simulink model "power"  (R2021a)
settings: Solver=VariableStepAuto  StartTime=0.0  StopTime=Torb  RelTol=1e-3
values from neighbouring files (symbols this model uses):
  inc = 97.5*pi/180    (= 1.70169602069)    [params_power.m]
libraries: sharedtransform x12, aerolibutil x4
settings Model: Creator=Laura  LastModifiedBy=Laura

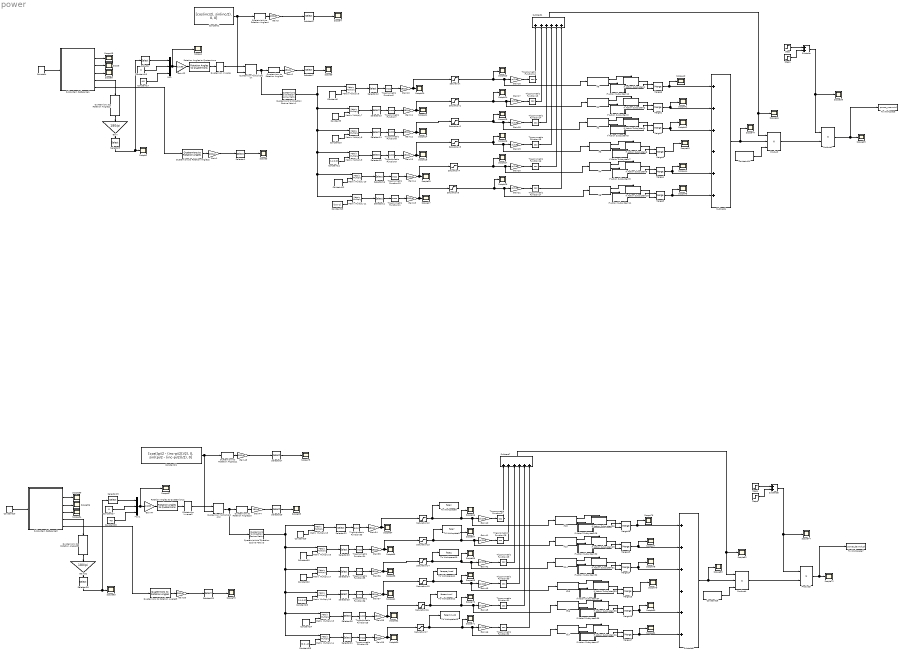
== system power ==
  Constant : Constant  Value=[0,0,0]
  Constant1 : Constant  Value=[cos(inc/2), sin(inc/2), 0, 0]
  Constant10 : Constant  Value=[0,0,1]
  Constant11 : Constant  Value=[-1,0,0]
  Constant12 : Constant  Value=[0,-1,0]
  Constant13 : Constant  Value=[0,0,-1]
  Constant14 : Constant  Value=1367*0.9*0.32*0.77
  Constant15 : Constant  Value=0
  Constant17 : Constant  Value=-45
  Constant20 : Constant  Value=[0,0,0]
  Constant21 : Constant  Value=[cos((pi/2 - (inc-pi/2))/2), 0, sin((pi/2 - (inc-pi/2))/2), 0]
  Constant22 : Constant  Value=[0,0,1]
  Constant23 : Constant  Value=[-1,0,0]
  Constant24 : Constant  Value=[0,-1,0]
  Constant25 : Constant  Value=[0,0,-1]
  Constant26 : Constant  Value=1367*0.9*0.32*0.77
  Constant27 : Constant  Value=0
  Constant28 : Constant  Value=-45
  Constant29 : Constant  Value=[1,0,0]
  Constant30 : Constant  Value=[0,1,0]
  Constant8 : Constant  Value=[1,0,0]
  Constant9 : Constant  Value=[0,1,0]
  Gain{,1..3,10..15,32..39,44,48} (20 alike) : Gain  Gain=180/pi
  Gain{16..22,40..43,45..47} (14 alike) : Gain  Gain=pi/180
  If Action Subsystem1 : Subsystem  TreatAsAtomicUnit=on
  If Action Subsystem10 : Subsystem  TreatAsAtomicUnit=on
  If Action Subsystem11 : Subsystem  TreatAsAtomicUnit=on
  If Action Subsystem12 : Subsystem  TreatAsAtomicUnit=on
  If Action Subsystem2 : Subsystem  TreatAsAtomicUnit=on
  If Action Subsystem25 : Subsystem  TreatAsAtomicUnit=on
  If Action Subsystem26 : Subsystem  TreatAsAtomicUnit=on
  If Action Subsystem27 : Subsystem  TreatAsAtomicUnit=on
  If Action Subsystem28 : Subsystem  TreatAsAtomicUnit=on
  If Action Subsystem29 : Subsystem  TreatAsAtomicUnit=on
  If Action Subsystem3 : Subsystem  TreatAsAtomicUnit=on
  If Action Subsystem30 : Subsystem  TreatAsAtomicUnit=on
  If Action Subsystem31 : Subsystem  TreatAsAtomicUnit=on
  If Action Subsystem32 : Subsystem  TreatAsAtomicUnit=on
  If Action Subsystem33 : Subsystem  TreatAsAtomicUnit=on
  If Action Subsystem34 : Subsystem  TreatAsAtomicUnit=on
  If Action Subsystem35 : Subsystem  TreatAsAtomicUnit=on
  If Action Subsystem36 : Subsystem  TreatAsAtomicUnit=on
  If Action Subsystem4 : Subsystem  TreatAsAtomicUnit=on
  If Action Subsystem5 : Subsystem  TreatAsAtomicUnit=on
  If Action Subsystem6 : Subsystem  TreatAsAtomicUnit=on
  If Action Subsystem7 : Subsystem  TreatAsAtomicUnit=on
  If Action Subsystem8 : Subsystem  TreatAsAtomicUnit=on
  If Action Subsystem9 : Subsystem  TreatAsAtomicUnit=on
  If{1..6,13..18} (12 alike) : If  IfExpression=u1 < 89.995
  Matrix Multiply{6..11,13..18} (12 alike) : Product  Multiplication=Matrix(*)
  Merge{1..6,13..18} (12 alike) : Merge
  Mux : Mux  Inputs=3
  Mux1 : Mux  Inputs=3
  Product : Product  Inputs=3
  Product1 : Product
  Product4 : Product  Inputs=3
  Product5 : Product
  Quaternion Inverse : aerolibutil/Quaternion Inverse
  Quaternion Inverse2 : aerolibutil/Quaternion Inverse
  Quaternion Multiplication : aerolibutil/Quaternion Multiplication
  Quaternion Multiplication2 : aerolibutil/Quaternion Multiplication
  Quaternions to Direction Cosine Matrix1 : sharedtransform/Quaternions to  Direction Cosine Matrix  aMode=aMode
      settings: SourceProductBaseCode=AE,PW,DR,MT,UV,VE
  Quaternions to Direction Cosine Matrix3 : sharedtransform/Quaternions to  Direction Cosine Matrix  aMode=aMode
      settings: SourceProductBaseCode=AE,PW,DR,MT,UV,VE
  Quaternions to Rotation Angles{1..5,9..11} (8 alike) : sharedtransform/Quaternions to Rotation Angles  rotationOrder=ZYX  aMode=aMode
      settings: SourceProductBaseCode=AE,PW,DR,MT,UV,VE
  Rotation Angles to Quaternions : sharedtransform/Rotation Angles to Quaternions  rotationOrder=ZYX  aMode=aMode
      settings: SourceProductBaseCode=AE,PW,DR,MT,UV,VE
  Rotation Angles to Quaternions1 : sharedtransform/Rotation Angles to Quaternions  rotationOrder=ZYX  aMode=aMode
      settings: SourceProductBaseCode=AE,PW,DR,MT,UV,VE
  Saturation{,1..5,12..17} (12 alike) : Saturate  UpperLimit=90.00005  LowerLimit=-90.00005
  Scope{,1..4,8..9,14..15,17..21,23..29,39..47,56..85} (60 alike) : Scope
  Selector : Selector  InputPortWidth=3  IndexOptions=Index vector (dialog)  Indices=[3]  OutputSizes=1
  Selector{1..3,7,20,27..29} (8 alike) : Selector  InputPortWidth=3  IndexOptions=Index vector (dialog)  Indices=[3 2 1]  OutputSizes=1
  Selector{11..16,21..26} (12 alike) : Selector  InputPortWidth=3  IndexOptions=Index vector (dialog)  Indices=[1]  OutputSizes=1
  Selector19 : Selector  InputPortWidth=3  IndexOptions=Index vector (dialog)  Indices=[3]  OutputSizes=1
  Step : Step  Time=30.76*60  Before=1  After=0  SampleTime=0
  Step1 : Step  Time=(30.76 + 35)*60  SampleTime=0
  Step4 : Step  Time=43.27*60  Before=1  After=0  SampleTime=0
  Step5 : Step  Time=(43.27 + 10)*60  SampleTime=0
  Subsystem Reference1 : Subsystem  ReferencedSubsystem=DKE_detumbling
  Subsystem Reference3 : Subsystem  ReferencedSubsystem=DKE_detumbling
  Subtract : Sum
  Subtract{1,4,7..8} (4 alike) : Sum  Inputs=++++++
  Subtract6 : Sum
  To Workspace : ToWorkspace  VariableName=power_noonmid  SaveFormat=Timeseries  SampleTime=-1
  To Workspace10 : ToWorkspace  VariableName=faceZ  SaveFormat=Timeseries  SampleTime=-1
  To Workspace11 : ToWorkspace  VariableName=facepayload  SaveFormat=Timeseries  SampleTime=-1
  To Workspace12 : ToWorkspace  VariableName=faceminusY  SaveFormat=Timeseries  SampleTime=-1
  To Workspace13 : ToWorkspace  VariableName=faceminusZ  SaveFormat=Timeseries  SampleTime=-1
  To Workspace7 : ToWorkspace  VariableName=power_dawndusk  SaveFormat=Timeseries  SampleTime=-1
  To Workspace8 : ToWorkspace  VariableName=faceX  SaveFormat=Timeseries  SampleTime=-1
  To Workspace9 : ToWorkspace  VariableName=faceY  SaveFormat=Timeseries  SampleTime=-1
  Trigonometric Function{6..11,25..26,33..36} (12 alike) : Trigonometry  Operator=acos
  Trigonometric Function{12..17,27..32} (12 alike) : Trigonometry  Operator=cos
  wires:
  Quaternions to Rotation Angles1/1 -> Gain/1
  Subsystem Reference1/3 -> Scope/1
  Subsystem Reference1/2 -> Scope15/1
  Subsystem Reference1/4 -> Scope8/1
  Subsystem Reference1/6 -> Quaternions to Rotation Angles2/1
  Gain/1 -> Selector3/1
  Constant/1 -> Subsystem Reference1/1
  Quaternions to Rotation Angles2/1 -> Gain1/1
  Constant1/1 -> Quaternions to Rotation Angles4/1, Quaternion Multiplication/2
  Gain2/1 -> Selector7/1
  Quaternions to Rotation Angles3/1 -> Gain2/1
  Quaternions to Rotation Angles4/1 -> Gain3/1
  Selector1/1 -> Scope3/1
  Gain1/1 -> Selector1/1
  Selector2/1 -> Scope4/1
  Gain3/1 -> Selector2/1
  Selector12/1 -> Trigonometric Function6/1
  Quaternion Multiplication/1 -> Quaternions to Direction Cosine Matrix1/1, Quaternions to Rotation Angles3/1
  Constant9/1 -> Matrix Multiply7/2
  Selector14/1 -> Trigonometric Function8/1
  Trigonometric Function7/1 -> Gain11/1
  Matrix Multiply6/1 -> Selector12/1
  Matrix Multiply11/1 -> Selector11/1
  Constant13/1 -> Matrix Multiply11/2
  Constant11/1 -> Matrix Multiply9/2
  Selector16/1 -> Trigonometric Function10/1
  Trigonometric Function11/1 -> Gain15/1
  Selector13/1 -> Trigonometric Function7/1
  Trigonometric Function10/1 -> Gain14/1
  Selector11/1 -> Trigonometric Function11/1
  Matrix Multiply9/1 -> Selector15/1
  Constant12/1 -> Matrix Multiply10/2
  Matrix Multiply10/1 -> Selector16/1
  Trigonometric Function8/1 -> Gain12/1
  Selector15/1 -> Trigonometric Function9/1
  Constant8/1 -> Matrix Multiply6/2
  Trigonometric Function9/1 -> Gain13/1
  Matrix Multiply7/1 -> Selector13/1
  Trigonometric Function6/1 -> Gain10/1
  Matrix Multiply8/1 -> Selector14/1
  Quaternions to Direction Cosine Matrix1/1 -> Matrix Multiply6/1, Matrix Multiply8/1, Matrix Multiply9/1, Matrix Multiply10/1, Matrix Multiply11/1, Matrix Multiply7/1
  Gain10/1 -> Saturation/1, Scope20/1  "X"
  Gain11/1 -> Saturation1/1, Scope21/1  "y"
  Gain12/1 -> Saturation2/1, Scope14/1  "Z"
  Gain13/1 -> Saturation3/1, Scope18/1  "payload"
  Gain14/1 -> Saturation4/1, Scope19/1  "-Y"
  Gain15/1 -> Saturation5/1, Scope17/1  "-Z"
  Saturation/1 -> If6/1, Gain16/1, Scope23/1  "Angles [deg] wrt sunlight. Noon-midnight"
  Saturation1/1 -> If1/1, Gain17/1, Scope24/1  "Angles [deg] wrt sunlight. Noon-midnight"
  Gain16/1 -> Trigonometric Function12/1
  Gain17/1 -> Trigonometric Function13/1
  Gain18/1 -> Trigonometric Function14/1
  Saturation2/1 -> If2/1, Gain18/1, Scope25/1  "Angles [deg] wrt sunlight. Noon-midnight"
  Gain19/1 -> Trigonometric Function15/1
  Saturation3/1 -> If3/1, Gain19/1, Scope26/1  "Angles [deg] wrt sunlight. Noon-midnight"
  Gain20/1 -> Trigonometric Function16/1
  Saturation4/1 -> Gain20/1, If4/1, Scope27/1  "Angles [deg] wrt sunlight. Noon-midnight"
  Gain21/1 -> Trigonometric Function17/1
  Saturation5/1 -> If5/1, Gain21/1, Scope28/1  "Angles [deg] wrt sunlight. Noon-midnight"
  Step/1 -> Subtract/1
  Subtract/1 -> Scope39/1, Product1/1
  Step1/1 -> Subtract/2
  Rotation Angles to Quaternions/1 -> Quaternion Inverse/1
  Selector3/1 -> Scope2/1, Selector/1
  Constant15/1 -> Mux/2
  Gain22/1 -> Rotation Angles to Quaternions/1
  Mux/1 -> Scope1/1, Gain22/1
  Subsystem Reference1/5 -> Quaternions to Rotation Angles1/1
  Quaternion Inverse/1 -> Quaternion Multiplication/1
  Selector/1 -> Mux/1
  Constant17/1 -> Mux/3
  Constant10/1 -> Matrix Multiply8/2
  Selector7/1 -> Scope9/1
  If Action Subsystem2/1(Out1) -> Merge1/2
  If1/1 -> If Action Subsystem2/Action
  If1/2 -> If Action Subsystem3/Action
  If Action Subsystem3/1(Out1) -> Merge1/1
  Merge1/1 -> Scope41/1, Subtract4/2
  Trigonometric Function13/1 -> Subtract1/2
  If Action Subsystem4/1(Out1) -> Merge2/2
  If2/2 -> If Action Subsystem5/Action
  Merge2/1 -> Subtract4/3, Scope42/1
  If2/1 -> If Action Subsystem4/Action
  If Action Subsystem5/1(Out1) -> Merge2/1
  Trigonometric Function14/1 -> Subtract1/3
  If Action Subsystem6/1(Out1) -> Merge3/2
  If3/2 -> If Action Subsystem7/Action
  Trigonometric Function15/1 -> Subtract1/4
  Merge3/1 -> Scope43/1
  If3/1 -> If Action Subsystem6/Action
  If Action Subsystem7/1(Out1) -> Merge3/1
  If4/1 -> If Action Subsystem8/Action
  If4/2 -> If Action Subsystem9/Action
  Merge4/1 -> Scope44/1, Subtract4/5
  If Action Subsystem9/1(Out1) -> Merge4/1
  Trigonometric Function16/1 -> Subtract1/5
  If Action Subsystem8/1(Out1) -> Merge4/2
  If5/1 -> If Action Subsystem10/Action
  If5/2 -> If Action Subsystem11/Action
  Merge5/1 -> Scope45/1, Subtract4/6
  If Action Subsystem11/1(Out1) -> Merge5/1
  Trigonometric Function17/1 -> Subtract1/6
  If Action Subsystem10/1(Out1) -> Merge5/2
  If6/1 -> If Action Subsystem1/Action
  If6/2 -> If Action Subsystem12/Action
  Merge6/1 -> Subtract4/1, Scope40/1
  If Action Subsystem12/1(Out1) -> Merge6/1
  Trigonometric Function12/1 -> Subtract1/1
  If Action Subsystem1/1(Out1) -> Merge6/2
  Subtract4/1 -> Scope47/1, Product/2
  Constant14/1 -> Product/3
  Subtract1/1 -> Scope46/1, Product/1
  Product/1 -> Product1/2
  Product1/1 -> To Workspace/1, Scope29/1
  Merge17/1 -> Scope81/1, Subtract8/6
  Matrix Multiply16/1 -> Selector23/1
  Gain46/1 -> Trigonometric Function32/1
  Gain41/1 -> Trigonometric Function28/1
  Quaternion Inverse2/1 -> Quaternion Multiplication2/1
  If Action Subsystem28/1(Out1) -> Merge18/1
  If13/2 -> If Action Subsystem30/Action
  If16/1 -> If Action Subsystem35/Action
  Quaternions to Rotation Angles11/1 -> Gain48/1
  If Action Subsystem35/1(Out1) -> Merge16/2
  Gain35/1 -> Saturation13/1, Scope65/1  "y"
  If18/2 -> If Action Subsystem28/Action
  If16/2 -> If Action Subsystem36/Action
  If18/1 -> If Action Subsystem25/Action
  If Action Subsystem36/1(Out1) -> Merge16/1
  If15/1 -> If Action Subsystem33/Action
  Selector23/1 -> Trigonometric Function34/1
  Gain48/1 -> Selector27/1
  If15/2 -> If Action Subsystem34/Action
  Trigonometric Function28/1 -> Subtract7/2
  If Action Subsystem34/1(Out1) -> Merge15/1
  Constant23/1 -> Matrix Multiply18/2
  Step5/1 -> Subtract6/2
  Saturation13/1 -> To Workspace9/1, If13/1, Gain41/1, Scope67/1  "Angles [deg] wrt sunlight. Dawn-dusk"
  Trigonometric Function31/1 -> Subtract7/5
  Trigonometric Function27/1 -> Subtract7/1
  Subsystem Reference3/4 -> Scope84/1
  If17/1 -> If Action Subsystem26/Action
  Mux1/1 -> Scope57/1, Gain47/1
  Constant30/1 -> Matrix Multiply16/2
  Quaternions to Rotation Angles9/1 -> Gain33/1
  Trigonometric Function34/1 -> Gain35/1
  Quaternions to Rotation Angles5/1 -> Gain32/1
  Subtract7/1 -> Scope82/1, Product4/1
  Rotation Angles to Quaternions1/1 -> Quaternion Inverse2/1
  If17/2 -> If Action Subsystem27/Action
  Quaternions to Rotation Angles10/1 -> Gain44/1
  Subtract8/1 -> Scope83/1, Product4/2
  If Action Subsystem32/1(Out1) -> Merge14/1
  Constant29/1 -> Matrix Multiply15/2
  Constant27/1 -> Mux1/2
  Constant24/1 -> Matrix Multiply13/2
  Trigonometric Function29/1 -> Subtract7/3
  If Action Subsystem27/1(Out1) -> Merge17/1
  Trigonometric Function30/1 -> Subtract7/4
  Merge15/1 -> Scope79/1
  Saturation14/1 -> To Workspace10/1, If14/1, Gain42/1, Scope68/1  "Angles [deg] wrt sunlight. Dawn-dusk"
  If Action Subsystem31/1(Out1) -> Merge14/2
  Gain45/1 -> Trigonometric Function31/1
  Merge14/1 -> Subtract8/3, Scope78/1
  If Action Subsystem26/1(Out1) -> Merge17/2
  If Action Subsystem33/1(Out1) -> Merge15/2
  Constant20/1 -> Subsystem Reference3/1
  If Action Subsystem25/1(Out1) -> Merge18/2
  If14/1 -> If Action Subsystem31/Action
  Merge18/1 -> Subtract8/1, Scope76/1
  Trigonometric Function32/1 -> Subtract7/6
  Selector26/1 -> Trigonometric Function25/1
  Selector29/1 -> Scope85/1
  If Action Subsystem29/1(Out1) -> Merge13/2
  If14/2 -> If Action Subsystem32/Action
  Quaternions to Direction Cosine Matrix3/1 -> Matrix Multiply15/1, Matrix Multiply17/1, Matrix Multiply18/1, Matrix Multiply13/1, Matrix Multiply14/1, Matrix Multiply16/1
  Constant26/1 -> Product4/3
  Merge13/1 -> Scope77/1, Subtract8/2
  If13/1 -> If Action Subsystem29/Action
  If Action Subsystem30/1(Out1) -> Merge13/1
  Selector19/1 -> Mux1/1
  Matrix Multiply17/1 -> Selector24/1
  Constant25/1 -> Matrix Multiply14/2
  Subsystem Reference3/5 -> Quaternions to Rotation Angles5/1
  Gain47/1 -> Rotation Angles to Quaternions1/1
  Constant22/1 -> Matrix Multiply17/2
  Subsystem Reference3/6 -> Quaternions to Rotation Angles9/1
  Selector25/1 -> Trigonometric Function36/1
  Saturation17/1 -> To Workspace13/1, If17/1, Gain46/1, Scope71/1  "Angles [deg] wrt sunlight. Dawn-dusk"
  Gain42/1 -> Trigonometric Function29/1
  Step4/1 -> Subtract6/1
  Trigonometric Function25/1 -> Gain38/1
  Constant28/1 -> Mux1/3
  Gain34/1 -> Saturation12/1, Scope64/1  "X"
  Selector21/1 -> Trigonometric Function26/1
  Selector24/1 -> Trigonometric Function35/1
  Matrix Multiply13/1 -> Selector26/1
  Trigonometric Function26/1 -> Gain39/1
  Gain38/1 -> Saturation16/1, Scope62/1  "-Y"
  Matrix Multiply18/1 -> Selector25/1
  Merge16/1 -> Scope80/1, Subtract8/5
  Gain36/1 -> Saturation14/1, Scope58/1  "Z"
  Trigonometric Function35/1 -> Gain36/1
  Gain43/1 -> Trigonometric Function30/1
  Trigonometric Function36/1 -> Gain37/1
  Saturation12/1 -> To Workspace8/1, If18/1, Gain40/1, Scope66/1  "Angles [deg] wrt sunlight. Dawn-dusk"
  Trigonometric Function33/1 -> Gain34/1
  Subtract6/1 -> Product5/1, Scope74/1
  Matrix Multiply14/1 -> Selector21/1
  Selector28/1 -> Scope63/1, Selector19/1
  Gain32/1 -> Selector28/1
  Saturation15/1 -> To Workspace11/1, If15/1, Gain43/1, Scope69/1  "Angles [deg] wrt sunlight. Dawn-dusk"
  Subsystem Reference3/2 -> Scope59/1
  Constant21/1 -> Quaternions to Rotation Angles11/1, Quaternion Multiplication2/2
  Quaternion Multiplication2/1 -> Quaternions to Direction Cosine Matrix3/1, Quaternions to Rotation Angles10/1
  Gain40/1 -> Trigonometric Function27/1
  Selector27/1 -> Scope75/1
  Saturation16/1 -> To Workspace12/1, Gain45/1, If16/1, Scope70/1  "Angles [deg] wrt sunlight. Dawn-dusk"
  Gain33/1 -> Selector20/1
  Gain39/1 -> Saturation17/1, Scope60/1  "-Z"
  Matrix Multiply15/1 -> Selector22/1
  Selector22/1 -> Trigonometric Function33/1
  Selector20/1 -> Scope73/1
  Gain44/1 -> Selector29/1
  Subsystem Reference3/3 -> Scope56/1
  Gain37/1 -> Saturation15/1, Scope61/1  "payload"
  Product4/1 -> Product5/2
  Product5/1 -> To Workspace7/1, Scope72/1

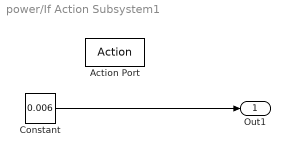
== system power/If Action Subsystem1 ==
  Action Port : ActionPort  ActionPortLabel=if(u1 < 89.995)
  Constant : Constant  Value=0.006
  Out1 : Outport
  wires:
  Constant/1 -> Out1/1

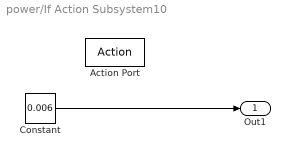
== system power/If Action Subsystem10 ==
  Action Port : ActionPort  ActionPortLabel=if(u1 < 89.995)
  Constant : Constant  Value=0.006
  Out1 : Outport
  wires:
  Constant/1 -> Out1/1

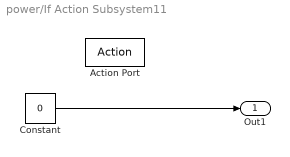
== system power/If Action Subsystem11 ==
  Action Port : ActionPort  ActionPortLabel=else
  Constant : Constant  Value=0
  Out1 : Outport
  wires:
  Constant/1 -> Out1/1

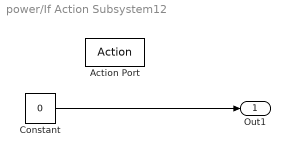
== system power/If Action Subsystem12 ==
  Action Port : ActionPort  ActionPortLabel=else
  Constant : Constant  Value=0
  Out1 : Outport
  wires:
  Constant/1 -> Out1/1

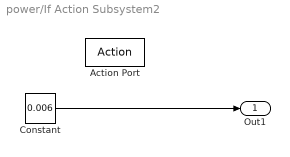
== system power/If Action Subsystem2 ==
  Action Port : ActionPort  ActionPortLabel=if(u1 < 89.995)
  Constant : Constant  Value=0.006
  Out1 : Outport
  wires:
  Constant/1 -> Out1/1

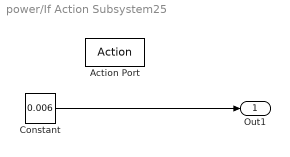
== system power/If Action Subsystem25 ==
  Action Port : ActionPort  ActionPortLabel=if(u1 < 89.995)
  Constant : Constant  Value=0.006
  Out1 : Outport
  wires:
  Constant/1 -> Out1/1

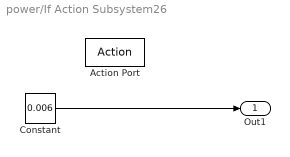
== system power/If Action Subsystem26 ==
  Action Port : ActionPort  ActionPortLabel=if(u1 < 89.995)
  Constant : Constant  Value=0.006
  Out1 : Outport
  wires:
  Constant/1 -> Out1/1

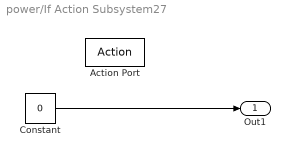
== system power/If Action Subsystem27 ==
  Action Port : ActionPort  ActionPortLabel=else
  Constant : Constant  Value=0
  Out1 : Outport
  wires:
  Constant/1 -> Out1/1

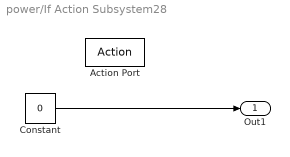
== system power/If Action Subsystem28 ==
  Action Port : ActionPort  ActionPortLabel=else
  Constant : Constant  Value=0
  Out1 : Outport
  wires:
  Constant/1 -> Out1/1

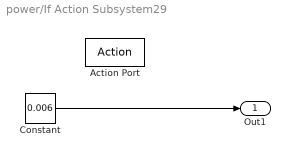
== system power/If Action Subsystem29 ==
  Action Port : ActionPort  ActionPortLabel=if(u1 < 89.995)
  Constant : Constant  Value=0.006
  Out1 : Outport
  wires:
  Constant/1 -> Out1/1

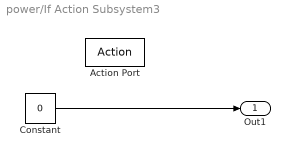
== system power/If Action Subsystem3 ==
  Action Port : ActionPort  ActionPortLabel=else
  Constant : Constant  Value=0
  Out1 : Outport
  wires:
  Constant/1 -> Out1/1

== system power/If Action Subsystem30 ==
  Action Port : ActionPort  ActionPortLabel=else
  Constant : Constant  Value=0
  Out1 : Outport
  wires:
  Constant/1 -> Out1/1

== system power/If Action Subsystem31 ==
  Action Port : ActionPort  ActionPortLabel=if(u1 < 89.995)
  Constant : Constant  Value=0.006
  Out1 : Outport
  wires:
  Constant/1 -> Out1/1

== system power/If Action Subsystem32 ==
  Action Port : ActionPort  ActionPortLabel=else
  Constant : Constant  Value=0
  Out1 : Outport
  wires:
  Constant/1 -> Out1/1

== system power/If Action Subsystem33 ==
  Action Port : ActionPort  ActionPortLabel=if(u1 < 89.995)
  Constant : Constant  Value=0.006
  Out1 : Outport
  wires:
  Constant/1 -> Out1/1

== system power/If Action Subsystem34 ==
  Action Port : ActionPort  ActionPortLabel=else
  Constant : Constant  Value=0
  Out1 : Outport
  wires:
  Constant/1 -> Out1/1

== system power/If Action Subsystem35 ==
  Action Port : ActionPort  ActionPortLabel=if(u1 < 89.995)
  Constant : Constant  Value=0.003
  Out1 : Outport
  wires:
  Constant/1 -> Out1/1

== system power/If Action Subsystem36 ==
  Action Port : ActionPort  ActionPortLabel=else
  Constant : Constant  Value=0
  Out1 : Outport
  wires:
  Constant/1 -> Out1/1

== system power/If Action Subsystem4 ==
  Action Port : ActionPort  ActionPortLabel=if(u1 < 89.995)
  Constant : Constant  Value=0.006
  Out1 : Outport
  wires:
  Constant/1 -> Out1/1

== system power/If Action Subsystem5 ==
  Action Port : ActionPort  ActionPortLabel=else
  Constant : Constant  Value=0
  Out1 : Outport
  wires:
  Constant/1 -> Out1/1

== system power/If Action Subsystem6 ==
  Action Port : ActionPort  ActionPortLabel=if(u1 < 89.995)
  Constant : Constant  Value=0.006
  Out1 : Outport
  wires:
  Constant/1 -> Out1/1

== system power/If Action Subsystem7 ==
  Action Port : ActionPort  ActionPortLabel=else
  Constant : Constant  Value=0
  Out1 : Outport
  wires:
  Constant/1 -> Out1/1

== system power/If Action Subsystem8 ==
  Action Port : ActionPort  ActionPortLabel=if(u1 < 89.995)
  Constant : Constant  Value=0.003
  Out1 : Outport
  wires:
  Constant/1 -> Out1/1

== system power/If Action Subsystem9 ==
  Action Port : ActionPort  ActionPortLabel=else
  Constant : Constant  Value=0
  Out1 : Outport
  wires:
  Constant/1 -> Out1/1
